simulink model "add_zeros"  (R2018a)
settings: Solver=VariableStepAuto  StartTime=0.0  StopTime=10.0  RelTol=1e-3
values from neighbouring files (symbols this model uses):
  b = 20e3    (= 20000)    [lab2.m]
  j = 600e3    (= 600000)    [lab2.m]
  k = 2000    [lab2.m]
settings Model: Creator=Mohamed Badr  LastModifiedBy=Mohamed Badr

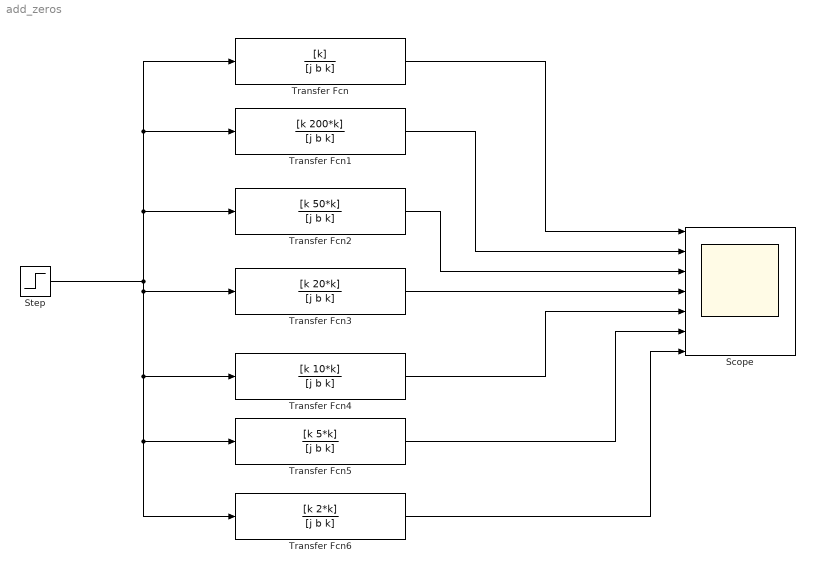
== system add_zeros ==
  Scope : Scope  NumInputPorts=7
  Step : Step  SampleTime=0
  Transfer Fcn : TransferFcn  Numerator=[k]  Denominator=[j b k]
  Transfer Fcn1 : TransferFcn  Numerator=[k 200*k]  Denominator=[j b k]
  Transfer Fcn2 : TransferFcn  Numerator=[k 50*k]  Denominator=[j b k]
  Transfer Fcn3 : TransferFcn  Numerator=[k 20*k]  Denominator=[j b k]
  Transfer Fcn4 : TransferFcn  Numerator=[k 10*k]  Denominator=[j b k]
  Transfer Fcn5 : TransferFcn  Numerator=[k 5*k]  Denominator=[j b k]
  Transfer Fcn6 : TransferFcn  Numerator=[k 2*k]  Denominator=[j b k]
  wires:
  Step/1 -> Transfer Fcn6/1, Transfer Fcn5/1, Transfer Fcn4/1, Transfer Fcn3/1, Transfer Fcn2/1, Transfer Fcn1/1, Transfer Fcn/1
  Transfer Fcn/1 -> Scope/1
  Transfer Fcn1/1 -> Scope/2
  Transfer Fcn2/1 -> Scope/3
  Transfer Fcn3/1 -> Scope/4
  Transfer Fcn4/1 -> Scope/5
  Transfer Fcn5/1 -> Scope/6
  Transfer Fcn6/1 -> Scope/7
